simulink model "lab9"  (R2023a)
settings: Solver=VariableStepAuto  StartTime=0.0  StopTime=10.0  RelTol=1e-3
libraries: simulink x3
settings Model: Creator=MUHAMMAD SADEEQ  LastModifiedBy=MUHAMMAD SADEEQ

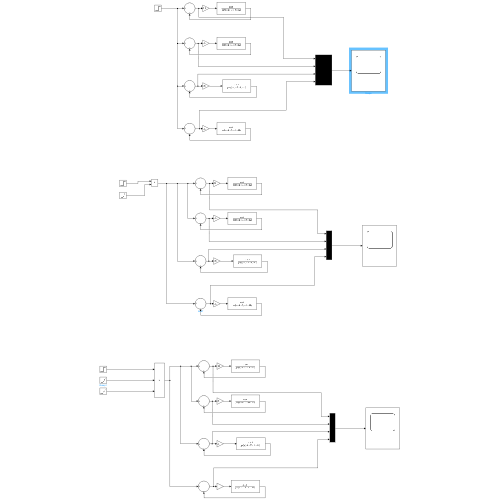
[thumbnail: Simulink's stored preview of the top-level diagram]
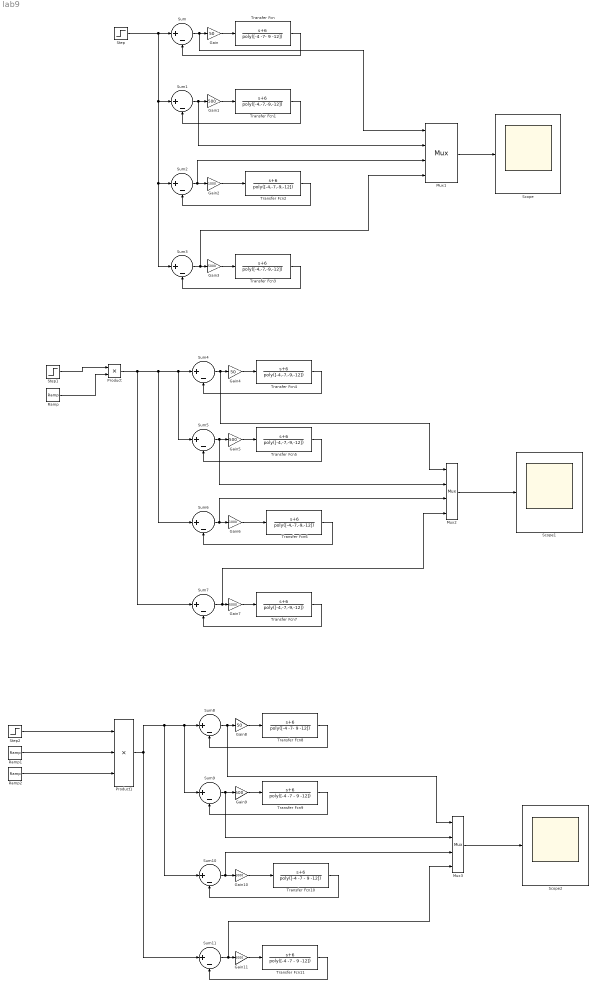
== system lab9 ==
  Gain : Gain  Gain=50
  Gain1 : Gain  Gain=500
  Gain10 : Gain  Gain=1000
  Gain11 : Gain  Gain=5000
  Gain2 : Gain  Gain=1000
  Gain3 : Gain  Gain=5000
  Gain4 : Gain  Gain=50
  Gain5 : Gain  Gain=500
  Gain6 : Gain  Gain=1000
  Gain7 : Gain  Gain=5000
  Gain8 : Gain  Gain=50
  Gain9 : Gain  Gain=500
  Mux1 : Mux
  Mux2 : Mux
  Mux3 : Mux
  Product : Product
  Product1 : Product  Inputs=3
  Ramp : simulink/Sources/Ramp  slope=1  start=0  InitialOutput=0
  Ramp1 : simulink/Sources/Ramp  slope=1  start=0  InitialOutput=0
  Ramp2 : simulink/Sources/Ramp  slope=1  start=0  InitialOutput=0
  Scope : Scope
  Scope1 : Scope
  Scope2 : Scope
  Step : Step  Time=0  After=5  SampleTime=0
  Step1 : Step  Time=0  After=5  SampleTime=0
  Step2 : Step  Time=0  After=5  SampleTime=0
  Sum{,1..11} (12 alike) : Sum  Inputs=|+-
  Transfer Fcn : TransferFcn  Numerator=[1,6]  Denominator=poly([-4 -7- 9 -12])
  Transfer Fcn{1..7} (7 alike) : TransferFcn  Numerator=[1,6]  Denominator=poly([-4,-7,-9,-12])
  Transfer Fcn10 : TransferFcn  Numerator=[1,6]  Denominator=poly([-4 -7 - 9 -12])
  Transfer Fcn11 : TransferFcn  Numerator=[1,6]  Denominator=poly([-4 -7 - 9 -12])
  Transfer Fcn8 : TransferFcn  Numerator=[1,6]  Denominator=poly([-4 -7- 9 -12])
  Transfer Fcn9 : TransferFcn  Numerator=[1,6]  Denominator=poly([-4 -7 - 9 -12])
  wires:
  Sum1/1 -> Mux1/2, Gain1/1
  Sum2/1 -> Mux1/3, Gain2/1
  Sum3/1 -> Mux1/4, Gain3/1
  Sum/1 -> Mux1/1, Gain/1
  Mux1/1 -> Scope/1
  Transfer Fcn/1 -> Sum/2
  Gain/1 -> Transfer Fcn/1
  Transfer Fcn1/1 -> Sum1/2
  Gain1/1 -> Transfer Fcn1/1
  Transfer Fcn3/1 -> Sum3/2
  Transfer Fcn2/1 -> Sum2/2
  Gain2/1 -> Transfer Fcn2/1
  Gain3/1 -> Transfer Fcn3/1
  Gain6/1 -> Transfer Fcn6/1
  Transfer Fcn5/1 -> Sum5/2
  Transfer Fcn7/1 -> Sum7/2
  Transfer Fcn6/1 -> Sum6/2
  Transfer Fcn4/1 -> Sum4/2
  Gain5/1 -> Transfer Fcn5/1
  Gain4/1 -> Transfer Fcn4/1
  Mux2/1 -> Scope1/1
  Sum7/1 -> Mux2/4, Gain7/1
  Gain7/1 -> Transfer Fcn7/1
  Sum5/1 -> Mux2/2, Gain5/1
  Sum6/1 -> Mux2/3, Gain6/1
  Sum4/1 -> Mux2/1, Gain4/1
  Product/1 -> Sum7/1, Sum6/1, Sum5/1, Sum4/1
  Step1/1 -> Product/1
  Ramp/1 -> Product/2
  Product1/1 -> Sum10/1, Sum9/1, Sum8/1, Sum11/1
  Gain9/1 -> Transfer Fcn9/1
  Sum11/1 -> Mux3/4, Gain11/1
  Sum9/1 -> Mux3/2, Gain9/1
  Sum8/1 -> Mux3/1, Gain8/1
  Gain8/1 -> Transfer Fcn8/1
  Mux3/1 -> Scope2/1
  Gain11/1 -> Transfer Fcn11/1
  Ramp1/1 -> Product1/2
  Sum10/1 -> Mux3/3, Gain10/1
  Transfer Fcn11/1 -> Sum11/2
  Transfer Fcn9/1 -> Sum9/2
  Step2/1 -> Product1/1
  Gain10/1 -> Transfer Fcn10/1
  Transfer Fcn8/1 -> Sum8/2
  Transfer Fcn10/1 -> Sum10/2
  Ramp2/1 -> Product1/3
  Step/1 -> Sum3/1, Sum2/1, Sum1/1, Sum/1
